simulink model "Converter_stable"  (R2021b)
settings: Solver=VariableStepAuto  StartTime=0.0  StopTime=1  FixedStep=Ts  MaxStep=Ts  RelTol=1e-3  EnableMultiTasking=on
PreLoadFcn:
  | Ts=5e-6;
  | deci=20;
InitFcn:
  | Ts=5e-6;
  | deci=20;
undefined symbols (not defined in the file): DiscIntNeverNeededParam, sps
libraries: powerlib_extras x6, spsFirstOrderFilterLib x5, spsThreePhaseSeriesRLCBranchLib x5, spsThreePhaseVIMeasurementLib x3, spsabctodq0Lib x3, spsGroundLib x3, spsSeriesRLCBranchLib x3, spsStairGeneratorLib x2, spsVoltageMeasurementLib x2, spsThreePhaseProgrammableVoltageSourceLib x2, dspsigops x1, spsdq0toabcLib x1
Description:
  | Copyright 2013-2015 Ruan Jiayang, Tsinghua Univ.
settings Model: Creator=XiaoLei  LastModifiedBy=Legend
settings DataIOCC: InitialState=xInit  LimitDataPoints=on  SaveFinalState=on  SaveFormat=StructureWithTime  SignalLoggingSaveFormat=ModelDataLogs  SaveOutput=off  SignalLogging=off  SaveTime=off  ReturnWorkspaceOutputs=off
settings OptimizationCC: ExpressionDepthLimit=2147483647  InitFltsAndDblsToZero=on  LifeSpan=inf
settings DebuggingCC: SaveWithParameterizedLinksMsg=none  UnderspecifiedInitializationDetection=Classic  MergeDetectMultiDrivingBlocksExec=none  SignalResolutionControl=TryResolveAllWithWarning  SolverPrmCheckMsg=warning  MultiTaskDSMMsg=warning  MultiTaskCondExecSysMsg=none  FcnCallInpInsideContextMsg=warning  UnconnectedInputMsg=none  UnconnectedOutputMsg=none  UnconnectedLineMsg=none  StateNameClashWarn=warning  SFUnexpectedBacktrackingDiag=warning  SFNoUnconditionalDefaultTransitionDiag=warning  SFMachineParentedDataDiag=warning  ArithmeticOperatorsInVariantConditions=warning
settings HardwareCC: ProdBitPerPointer=32  ProdBitPerSizeT=32  ProdBitPerPtrDiffT=32  ProdLargestAtomicFloat=None  ProdIntDivRoundTo=Undefined  ProdEndianess=Unspecified  ProdWordSize=32  ProdHWDeviceType=32-bit Generic
settings ModelReferenceCC: PropagateSignalLabelsOutOfModel=off
settings SFSimCC: SimUseLocalCustomCode=off  SimParseCustomCode=off  CustomCodeUndefinedFunction=UseInterfaceOnly
settings RTWCC: RTWUseLocalCustomCode=off
settings CodeAppCC: StateflowObjectComments=on
settings GRTTargetCC: TargetFcnLib=ansi_tfl_tmw.mat  TargetLangStandard=C89/C90 (ANSI)  CombineOutputUpdateFcns=off  GRTInterface=on
settings ConfigComp: CovMetricSettings=dw  CovSaveCumulativeToWorkspaceVar=on  CovSaveSingleToWorkspaceVar=on  CovExternalEMLEnable=off
settings SimscapeCC: SimscapeNormalizeSystem=off

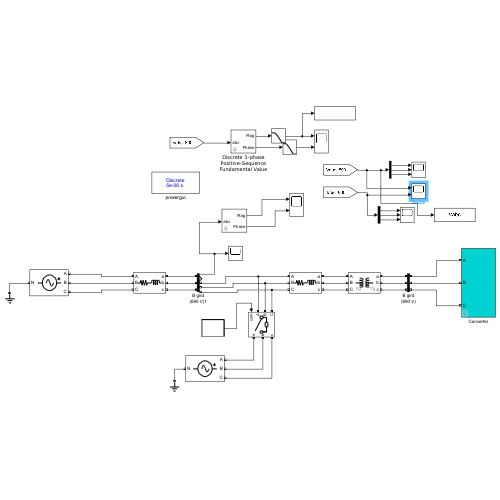
[thumbnail: Simulink's stored preview of the top-level diagram]
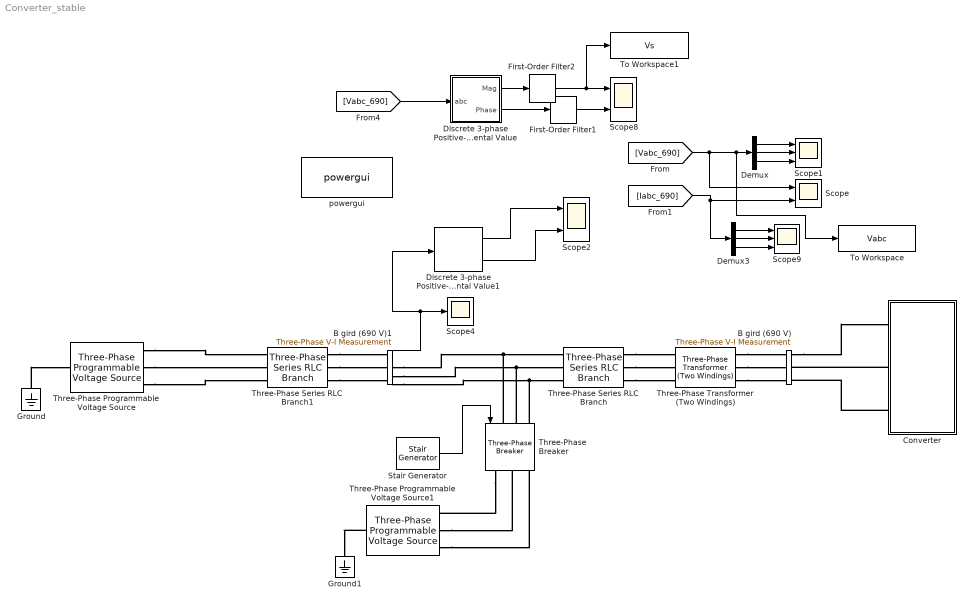
== system Converter_stable ==
  B gird (690 V) : spsThreePhaseVIMeasurementLib/Three-Phase V-I Measurement  VoltageMeasurement=phase-to-ground  SetLabelV=on  LabelV=Vabc_690  Vpu=on  VpuLL=off  CurrentMeasurement=yes  SetLabelI=on  LabelI=Iabc_690  Ipu=on  Pbase=0.5e6*0.9  Vbase=380  OutputType=Complex  PhasorSimulation=off  PSBequivalent=0
  B gird (690 V)1 : spsThreePhaseVIMeasurementLib/Three-Phase V-I Measurement  VoltageMeasurement=phase-to-ground  SetLabelV=off  LabelV=Vabc_690  Vpu=on  VpuLL=off  CurrentMeasurement=yes  SetLabelI=off  LabelI=Iabc_690  Ipu=on  Pbase=0.5e6  Vbase=10e3  OutputType=Complex  PhasorSimulation=off  PSBequivalent=0
  Converter : Subsystem  mask{Nb_wt=1, Vnom=690, Pnom1=1.5e6, Fnom=50, RL_grid=[0.01 0.25], CDC_link1=10000e-6*5, Vdc_nom=1200, Np=123, Fb_time_const=0.005, K1=[15 25 15 50/2], K2=[40 500 2 10], K3=[0.5 15], K4=0}
      mask prompts: Nb_wt "Number of wind turbines"; Vnom "Rated L-L Voltage(V)"; Pnom1 "Rated Power(VA)"; Fnom "Rated Frequency(Hz)"; RL_grid "Grid-side coupling impedance(p.u.)"; CDC_link1 "DC bus capitance (F)"; Vdc_nom "DC capacitor voltage(V)"; Np "Number of pole pairs"; Fb_time_const "Feed back time constant(s)"; K1 "rotor-side Id & Iq PID"; K2 "grid-side Vdc & Vdq PID"; K3 "rotor-side Pm PID"; K4 "gird-side Qref PID"
      mask init:
      | R_RL=RL_grid(1);
      | L_RL=RL_grid(2);
      | CDC_link=CDC_link1*Nb_wt;
      | Pnom=Pnom1*Nb_wt;
      | Inom=Pnom/sqrt(3)/Vnom;
      | Znom=Vnom/sqrt(3)/Inom;
      | Lnom=Znom/2/pi/Fnom;
      | Flux_nom=sqrt(2/3)*Vnom/2/pi/Fnom;
      | Rs_pu= 0.0034;
      | Ldq_pu= 0.352;
      | Rs=Rs_pu*Znom
      | Ldq=Ldq_pu*Lnom
      | Flux_pu=1.0017;
      | % H=0.685+4.32;
      | J_pu=0.1427/5;
      | Jnom=(2*pi*Fnom/Np)^(-2)*Pnom;
      | J=J_pu*Jnom;
      | % J=35000;%(2*pi*Fnom/Np)^(-2)*2*H*Pnom
      | Flux=Flux_pu*Flux_nom;
      | Vw_rated=11;%额定风速
      | Wr_rated=2.55;%额定转速
      | Radius=sqrt(Pnom1*2/1.225/pi/0.48/Vw_rated^3) %1.1225 is the air density, 0.44 is the maximum wind conversion rate
      | Kratio=8.119*Vw_rated/Radius/Wr_rated; %8.119 is the optimal  tip speed ratio
  Demux : Demux  Outputs=3
  Demux3 : Demux  Outputs=3
  Discrete 3-phase Positive-Sequence Fundamental Value : Subsystem  AncestorBlock=|  DialogController=POWERSYS.PowerSysDialog  mask(Discrete 3-phase Positive-sequence fundamental value){Freq=50, Par_Init=[0 0], Ts=Ts}
      | powerlib_extras/Discrete
      | Measurements/Discrete 3-phase
      | Positive-Sequence
      | Fundamental Value
      mask prompts: Freq "Fundamental frequency (Hz):"; Par_Init "Initial input (positive component): [ Mag  Phase(degrees) ]"; Ts "Sample time:"
      mask help:
      | Compute the positive-sequence component of the input signal at the given fundamental frequency. The input is set of three balanced or unbalanced signals which may contain harmonics.
      |
      | The two outputs return respectively the magnitude (same units as the input signal) and phase (in degrees) of the fundamental.
      |
      | For the first cycle of simulation, the outputs are held constant to the values specified by the Initial input parameter.
      mask init:
      | SamplesPerCycle=1/Freq/Ts;
      | RoundSamplesPerCycle=round(SamplesPerCycle);
      | Delay=RoundSamplesPerCycle*Ts - Ts/2;
      | Correction=SamplesPerCycle/RoundSamplesPerCycle - 1;
      | Real_Init=Par_Init(1)*cos(pi/180*Par_Init(2));
      | Imag_Init=Par_Init(1)*sin(pi/180*Par_Init(2));
      | power_initmask();
      mask Help: This block is part of a subset of blocks in the Extras library that does not have documentation associated with it, other than the block mask description.
      mask Display: disp('')
  Discrete 3-phase Positive-Sequence Fundamental Value1 : powerlib_extras/Discrete Measurements/Discrete 3-phase Positive-Sequence Fundamental Value  Freq=50  Par_Init=[0 0]  Ts=Ts
      settings: SourceProductBaseCode=PS
  First-Order Filter1 : spsFirstOrderFilterLib/First-Order Filter  FilterType=Lowpass  Tc=10e-3  Ts=0  Initialize=on  Vac_Init=[0, 0, 60]  Vdc_Init=0  PlotResponse=off  FreqRange="[0,  200,  1]"
  First-Order Filter2 : spsFirstOrderFilterLib/First-Order Filter  FilterType=Lowpass  Tc=5e-4  Ts=0  Initialize=on  Vac_Init=[0, 0, 60]  Vdc_Init=0  PlotResponse=off  FreqRange="[0,  200,  1]"
  Ground : spsGroundLib/Ground  LConnTagsString=a
  Ground1 : spsGroundLib/Ground  LConnTagsString=a
  Scope : Scope  NumInputPorts=2
  Scope1 : Scope  NumInputPorts=3
  Scope2 : Scope  NumInputPorts=2
  Scope4 : Scope
  Scope8 : Scope  NumInputPorts=2
  Scope9 : Scope  NumInputPorts=3
  Stair Generator : spsStairGeneratorLib/Stair Generator  t=[0, 0.6, 1.225]  e="[0, 1,  0]"  Ts=0
  Three-Phase Programmable Voltage Source : spsThreePhaseProgrammableVoltageSourceLib/Three-Phase Programmable Voltage Source  PositiveSequence=[10e3 0 50]  VariationEntity=None  VariationType=Table of time-amplitude pairs  VariationTypeAlt=Step  VariationStep=0.5  VariationRate=10  VariationMagnitude=0.3  VariationFrequency=2  VariationTiming=[1 2]  VariationPhaseA=off  Amplitudes=[1 0.15 1.0]  TimeValues=[0 0.6 2]  HarmonicGeneration=off  HarmonicA=[3 0.2 -25 0]  HarmonicB=[2 0.15 35 2]  Timing="[0.05  3]"  BusType=swing  Pref=0  Qref=0  Qmin=-inf  Qmax=inf
  Three-Phase Programmable Voltage Source1 : spsThreePhaseProgrammableVoltageSourceLib/Three-Phase Programmable Voltage Source  PositiveSequence=[0.2*10e3 -90 50]  VariationEntity=None  VariationType=Table of time-amplitude pairs  VariationTypeAlt=Step  VariationStep=0.5  VariationRate=10  VariationMagnitude=0.3  VariationFrequency=2  VariationTiming=[1 2]  VariationPhaseA=off  Amplitudes=[1 0.15 1.0]  TimeValues=[0 0.6 2]  HarmonicGeneration=off  HarmonicA=[3 0.2 -25 0]  HarmonicB=[2 0.15 35 2]  Timing="[0.05  3]"  BusType=swing  Pref=0  Qref=0  Qmin=-inf  Qmax=inf
  Three-Phase Series RLC Branch : spsThreePhaseSeriesRLCBranchLib/Three-Phase Series RLC Branch  LConnTagsString=A|B|C  RConnTagsString=A|B|C  BranchType=RL  Resistance=0.1*10*10/0.5  Inductance=0.33*10*10/0.5/314  Capacitance=1e-6  Measurements=None
  Three-Phase Series RLC Branch1 : spsThreePhaseSeriesRLCBranchLib/Three-Phase Series RLC Branch  LConnTagsString=A|B|C  RConnTagsString=A|B|C  BranchType=RL  Resistance=0.015*10*10/0.5  Inductance=0.15*10*10/0.5/314  Capacitance=1e-6  Measurements=None
  Three-Phase Transformer (Two Windings) : spsThreePhaseTransformerTwoWindingsLib/Three-Phase Transformer (Two Windings)  Winding1Connection=Yg  Winding2Connection=Yg  CoreType=Three single-phase transformers  SetSaturation=off  Hysteresis=off  DataFile='hysteresis'  SetInitialFlux=off  Measurements=None  UNITS=pu  NominalPower=[ 0.5e6 , 50 ]  Winding1=[ 10.5e3 , 0.0002 , 0.01 ]  Winding2=[ 0.38e3 , 0.0002 , 0.01 ]  Rm=500  Lm=500  L0=0.5  Saturation=[ 0,0 ; 0.0024,1.2 ; 1.0,1.52 ]  InitialFluxes=[ 0.8 , -0.8 , 0.7 ]  BreakLoop=off  DiscreteSolver=Trapezoidal iterative  DataType=off  TransfoNumber=1
  Three-Phase Breaker : spsThreePhaseBreakerLib/Three-Phase Breaker  InitialState=open  SwitchA=on  SwitchB=on  SwitchC=on  SwitchTimes="[1/60  5/60]"  External=on  BreakerResistance=0.00001  SnubberResistance=1e6  SnubberCapacitance=inf  Measurements=None
  To Workspace : ToWorkspace  VariableName=Vabc  SaveFormat=Timeseries  SampleTime=-1
  To Workspace1 : ToWorkspace  VariableName=Vs  SaveFormat=Timeseries  SampleTime=-1
  powergui : spspowerguiLib/powergui  SimulationMode=Discrete  SampleTime=Ts  frequency=50  Iterations=50  frequencyindice=0  Pbase=100e6  ErrMax=1e-4  UnitsV=kV  UnitsW=MW  buscounter=0  FunctionMessages=off  echomessages=off  EnableUseOfTLC=off  CurrentSourceSwitches=off  DisableSnubberDevices=off  DisableRonSwitches=off  DisableVfSwitches=off  DisplayEquations=off  AutomaticDiscreteSolvers=off  SolverType=Tustin/Backward Euler (TBE)  Interpol=off  ExternalGateDelay=off  methode=off  Ts=0  x0status=blocks  SPID=off  SwTol=0  HookPort=off  NonlinearTolerance=1e-4  nMaxIteration=100  ContinueOnMaxIteration=off  RestoreLinks=warning  ResistiveCurrentMeasurement=off  Frange=[0:2:500]  Ylog=off  Xlog=on  ShowGrid=off  save=off  variable=ZData  structure=Isabc  ZoomFFT=off  StartTime=1.29  cycles=2  DisplayStyle=1  fundamental=50  FreqAxis=off  MaxFrequency=1000  frequencyindicesteady=1  RmsSteady=1  display=off
  wires:
  [Vabc_690] -> Scope/1, To Workspace/1, Demux/1
  Demux/1 -> Scope1/1
  Demux/2 -> Scope1/2
  Demux/3 -> Scope1/3
  [Vabc_690] -> Discrete 3-phase Positive-Sequence Fundamental Value/1(abc)
  Discrete 3-phase Positive-Sequence Fundamental Value/2(Phase) -> First-Order Filter1/1
  Demux3/3 -> Scope9/3
  Demux3/2 -> Scope9/2
  Demux3/1 -> Scope9/1
  [Iabc_690] -> Demux3/1, Scope/2
  B gird (690 V)1/1 -> Scope4/1, Discrete 3-phase Positive-Sequence Fundamental Value1/1
  Discrete 3-phase Positive-Sequence Fundamental Value1/2 -> Scope2/2
  Discrete 3-phase Positive-Sequence Fundamental Value1/1 -> Scope2/1
  Stair Generator/1 -> Three-Phase Breaker/1
  Discrete 3-phase Positive-Sequence Fundamental Value/1(Mag) -> First-Order Filter2/1
  First-Order Filter1/1 -> Scope8/2
  First-Order Filter2/1 -> To Workspace1/1, Scope8/1
  connections:
  B gird (690 V)/RConn1 -- Converter/LConn1
  Converter/LConn2 -- B gird (690 V)/RConn2
  Converter/LConn3 -- B gird (690 V)/RConn3
  Ground/LConn1 -- Three-Phase Programmable Voltage Source/LConn1
  Three-Phase Series RLC Branch/RConn1 -- Three-Phase Transformer (Two Windings)/LConn1
  Three-Phase Series RLC Branch/RConn2 -- Three-Phase Transformer (Two Windings)/LConn2
  Three-Phase Series RLC Branch/RConn3 -- Three-Phase Transformer (Two Windings)/LConn3
  B gird (690 V)1/RConn1 -- Three-Phase Breaker/LConn1 -- Three-Phase Series RLC Branch/LConn1
  B gird (690 V)1/RConn2 -- Three-Phase Breaker/LConn2 -- Three-Phase Series RLC Branch/LConn2
  B gird (690 V)1/RConn3 -- Three-Phase Breaker/LConn3 -- Three-Phase Series RLC Branch/LConn3
  Three-Phase Programmable Voltage Source/RConn1 -- Three-Phase Series RLC Branch1/LConn1
  Three-Phase Programmable Voltage Source/RConn2 -- Three-Phase Series RLC Branch1/LConn2
  Three-Phase Programmable Voltage Source/RConn3 -- Three-Phase Series RLC Branch1/LConn3
  Three-Phase Transformer (Two Windings)/RConn1 -- B gird (690 V)/LConn1
  Three-Phase Transformer (Two Windings)/RConn2 -- B gird (690 V)/LConn2
  Three-Phase Transformer (Two Windings)/RConn3 -- B gird (690 V)/LConn3
  Three-Phase Series RLC Branch1/RConn1 -- B gird (690 V)1/LConn1
  Three-Phase Series RLC Branch1/RConn2 -- B gird (690 V)1/LConn2
  Three-Phase Series RLC Branch1/RConn3 -- B gird (690 V)1/LConn3
  Three-Phase Programmable Voltage Source1/RConn2 -- Three-Phase Breaker/RConn2
  Three-Phase Breaker/RConn1 -- Three-Phase Programmable Voltage Source1/RConn1
  Three-Phase Programmable Voltage Source1/RConn3 -- Three-Phase Breaker/RConn3
  Three-Phase Programmable Voltage Source1/LConn1 -- Ground1/LConn1

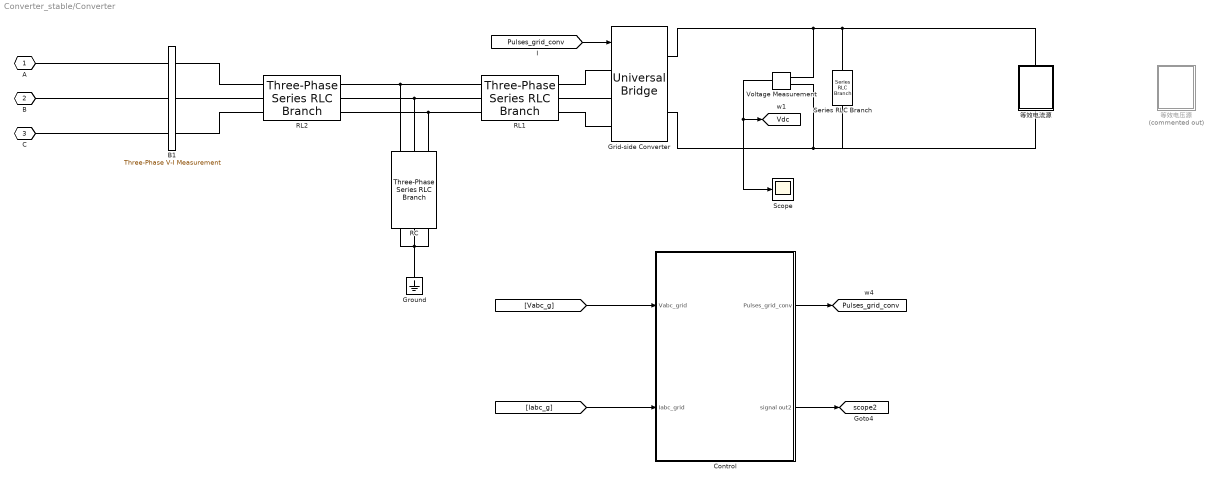
== system Converter_stable/Converter ==
  B1 : spsThreePhaseVIMeasurementLib/Three-Phase V-I Measurement  VoltageMeasurement=phase-to-ground  SetLabelV=on  LabelV=Vabc_g  Vpu=on  VpuLL=off  CurrentMeasurement=yes  SetLabelI=on  LabelI=Iabc_g  Ipu=on  Pbase=0.5e6  Vbase=380  OutputType=Complex  PhasorSimulation=off  PSBequivalent=0
  Control : Subsystem
  Grid-side Converter : spsUniversalBridgeLib/Universal Bridge  Arms=3  SnubberResistance=1e6  SnubberCapacitance=inf  Device=IGBT / Diodes  Ron=1e-7  Lon=0  ForwardVoltages="[  0  0  ]"  ForwardVoltage=0  GTOparameters=[ 10e-6 , 20e-6 ]  IGBTparameters=[0 , 0]  Measurements=None  Measurements_2=None  converterType=Rectifier
  Ground : spsGroundLib/Ground  LConnTagsString=a
  RC : spsThreePhaseSeriesRLCBranchLib/Three-Phase Series RLC Branch  LConnTagsString=A|B|C  RConnTagsString=A|B|C  BranchType=RC  Resistance=1.5  Inductance=L_RL*Vnom^2/Pnom/(2*pi*Fnom)  Capacitance=1000e-6  Measurements=None
  RL1 : spsThreePhaseSeriesRLCBranchLib/Three-Phase Series RLC Branch  LConnTagsString=A|B|C  RConnTagsString=A|B|C  BranchType=RL  Resistance=0.0002  Inductance=0.7/1000  Capacitance=1.0  Measurements=None
  RL2 : spsThreePhaseSeriesRLCBranchLib/Three-Phase Series RLC Branch  LConnTagsString=A|B|C  RConnTagsString=A|B|C  BranchType=RL  Resistance=0.0001  Inductance=0.3/1000  Capacitance=1.0  Measurements=None
  Scope : Scope
  Series RLC Branch : spsSeriesRLCBranchLib/Series RLC Branch  LConnTagsString=__new0  RConnTagsString=__new0  BranchType=C  Resistance=1  Inductance=1e-3  SetiL0=off  InitialCurrent=0  Capacitance=10000e-6  Setx0=on  InitialVoltage=790  Measurements=None
  Voltage Measurement : spsVoltageMeasurementLib/Voltage Measurement  PhasorSimulation=off  OutputType=Complex  PSBequivalent=0
  等效电压源 : Subsystem  Commented=on
  等效电流源 : Subsystem
  A : PMIOPort  Tag=PMCPort  Side=Left
  B : PMIOPort  Tag=PMCPort  Port=2  Side=Left
  C : PMIOPort  Tag=PMCPort  Port=3  Side=Left
  tag scope: Pulses_grid_conv=global, Vdc=global, scope2=global
  wires:
  [Pulses_grid_conv] -> Grid-side Converter/1
  Control/1(Pulses_grid_conv) -> [Pulses_grid_conv]
  Control/2(signal out2) -> [scope2]
  [Vabc_g] -> Control/1(Vabc_grid)
  [Iabc_g] -> Control/2(Iabc_grid)
  Voltage Measurement/1 -> Scope/1, [Vdc]
  connections:
  RL1/RConn1 -- Grid-side Converter/LConn1
  RL1/RConn2 -- Grid-side Converter/LConn2
  RL1/RConn3 -- Grid-side Converter/LConn3
  C/RConn1 -- B1/LConn3
  B1/LConn1 -- A/RConn1
  B1/LConn2 -- B/RConn1
  Ground/LConn1 -- RC/RConn2 -- RC/RConn3 -- RC/RConn1
  B1/RConn1 -- RL2/LConn1
  B1/RConn2 -- RL2/LConn2
  B1/RConn3 -- RL2/LConn3
  RL2/RConn1 -- RL1/LConn1 -- RC/LConn1
  RL2/RConn2 -- RL1/LConn2 -- RC/LConn2
  RL2/RConn3 -- RC/LConn3 -- RL1/LConn3
  Series RLC Branch/LConn1 -- 等效电流源/RConn1 -- Voltage Measurement/LConn1 -- Grid-side Converter/RConn1
  Grid-side Converter/RConn2 -- 等效电流源/LConn1 -- Series RLC Branch/RConn1 -- Voltage Measurement/LConn2

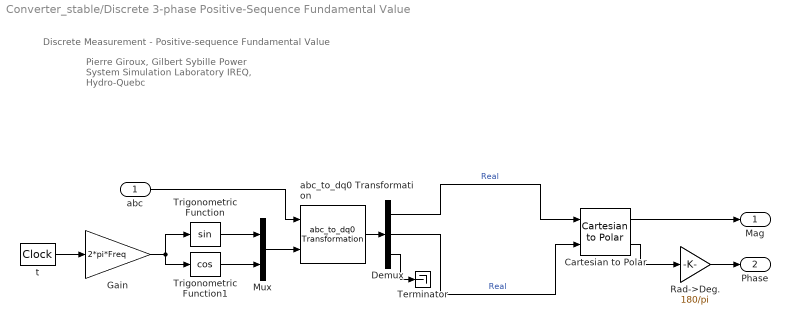
== system Converter_stable/Discrete 3-phase Positive-Sequence Fundamental Value ==
  note: Pierre Giroux, Gilbert Sybille
      | Power System Simulation Laboratory
      | IREQ, Hydro-Quebc
  note: Discrete Measurement - Positive-sequence Fundamental Value
  abc : Inport  PortDimensions=3
  Cartesian to Polar : simulink_extras/Transformations/Cartesian to Polar
  Demux : Demux  Outputs=3
      settings: DisplayOption=none
  Gain : Gain  Gain=2*pi*Freq  SaturateOnIntegerOverflow=on  OutDataTypeStr=Inherit: Same as input  ParamDataTypeStr=Inherit: Same as input
  Mux : Mux  Inputs=2
  Rad->Deg. : Gain  Gain=180/pi  SaturateOnIntegerOverflow=on  OutDataTypeStr=Inherit: Same as input  ParamDataTypeStr=Inherit: Same as input
  Terminator : Terminator
  Trigonometric Function : Trigonometry
  Trigonometric Function1 : Trigonometry  Operator=cos
  abc_to_dq0 Transformation : powerlib_extras/Measurements/abc_to_dq0 Transformation
      settings: SourceProductBaseCode=PS
  t : DigitalClock  SampleTime=Ts
  Mag : Outport  VectorParamsAs1DForOutWhenUnconnected=off
  Phase : Outport  Port=2  VectorParamsAs1DForOutWhenUnconnected=off
  wires:
  Cartesian to Polar/2 -> Rad->Deg./1
  Cartesian to Polar/1 -> Mag/1
  Gain/1 -> Trigonometric Function1/1, Trigonometric Function/1
  t/1 -> Gain/1
  abc/1 -> abc_to_dq0 Transformation/1
  Mux/1 -> abc_to_dq0 Transformation/2
  Demux/1 -> Cartesian to Polar/1  "Real"
  Rad->Deg./1 -> Phase/1
  Demux/2 -> Cartesian to Polar/2  "Real"
  abc_to_dq0 Transformation/1 -> Demux/1
  Demux/3 -> Terminator/1
  Trigonometric Function/1 -> Mux/1
  Trigonometric Function1/1 -> Mux/2

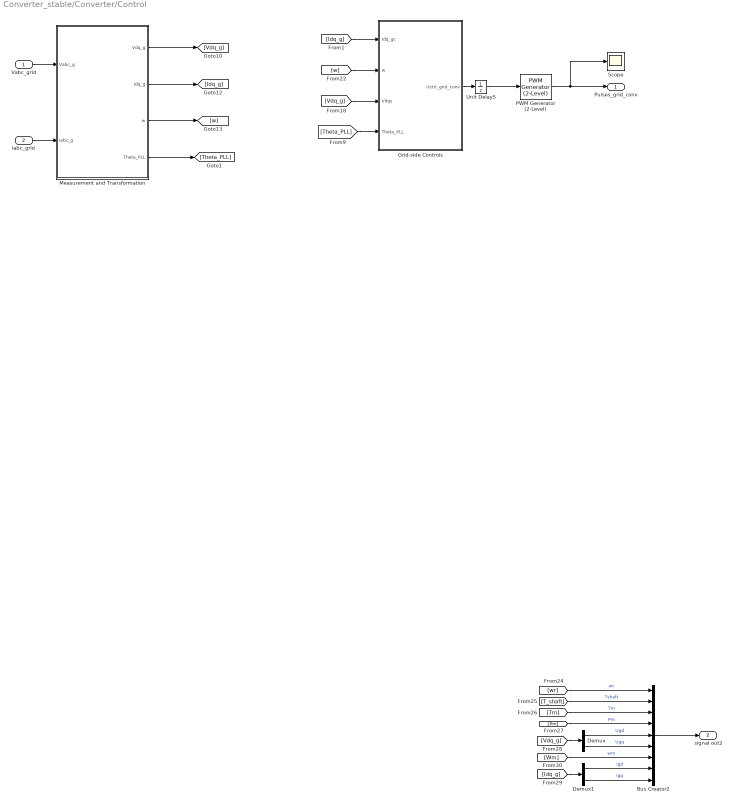
== system Converter_stable/Converter/Control ==
  Vabc_grid : Inport
  Iabc_grid : Inport  Port=2
  Bus Creator2 : BusCreator  Inputs=9
  Demux : Demux  Outputs=2
  Demux1 : Demux  Outputs=2
  Grid-side Controls : Subsystem
  Measurement and Transformation : Subsystem
  PWM Generator (2-Level) : spsPWMGenerator2LevelLib/PWM Generator (2-Level)  ModulatorType=Three-phase bridge (6 pulses)  ModulatorMode=Unsynchronized  Fc=3000  Pc=90  nF=27  MinMax="[ -1  1 ]"  SamplingTechnique=Natural  ModulatingSignals=off  m=0.8  Freq=60  Phase=0  Ts=Ts  ShowCarrierOutport=off
  Scope : Scope
  Unit Delay5 : UnitDelay  SampleTime=Ts  HasFrameUpgradeWarning=on
  Pulses_grid_conv : Outport
  signal out2 : Outport  Port=2
  wires:
  Measurement and Transformation/3(w) -> [w]
  Measurement and Transformation/2(Idq_g) -> [Idq_g]
  Measurement and Transformation/1(Vdq_g) -> [Vdq_g]
  Iabc_grid/1 -> Measurement and Transformation/2(Iabc_g)
  Vabc_grid/1 -> Measurement and Transformation/1(Vabc_g)
  Measurement and Transformation/4(Theta_PLL) -> [Theta_PLL]
  [Vdq_g] -> Grid-side Controls/3(Vdqs)
  [w] -> Grid-side Controls/2(w)
  [Idq_g] -> Grid-side Controls/1(Idq_gc)
  [Theta_PLL] -> Grid-side Controls/4(Theta_PLL)
  [wr] -> Bus Creator2/1  "wr"
  [T_shaft] -> Bus Creator2/2  "Tshaft"
  [Tm] -> Bus Creator2/3  "Tm"
  [Pm] -> Bus Creator2/4  "Pm"
  Bus Creator2/1 -> signal out2/1
  [Wm] -> Bus Creator2/7  "wm"
  [Vdq_g] -> Demux/1
  [Idq_g] -> Demux1/1
  Demux/1 -> Bus Creator2/5  "Ugd"
  Demux/2 -> Bus Creator2/6  "Ugq"
  Demux1/1 -> Bus Creator2/8  "Igd"
  Demux1/2 -> Bus Creator2/9  "Igq"
  Grid-side Controls/1(Uctrl_grid_conv) -> Unit Delay5/1
  Unit Delay5/1 -> PWM Generator (2-Level)/1
  PWM Generator (2-Level)/1 -> Pulses_grid_conv/1, Scope/1

== system Converter_stable/Converter/等效电压源 ==
  DC Voltage Source : spsDCVoltageSourceLib/DC Voltage Source  Amplitude=790  Measurements=None
  Series RLC Branch1 : spsSeriesRLCBranchLib/Series RLC Branch  LConnTagsString=__new0  RConnTagsString=__new0  BranchType=R  Resistance=0.01  Inductance=1e-3  SetiL0=off  InitialCurrent=0  Capacitance=5000e-6  Setx0=on  InitialVoltage=790  Measurements=None
  Conn1 : PMIOPort  Side=Right
  - : PMIOPort  Port=2  Side=Left
  connections:
  Series RLC Branch1/LConn1 -- DC Voltage Source/RConn1
  DC Voltage Source/LConn1 -- -/RConn1
  Series RLC Branch1/RConn1 -- Conn1/RConn1

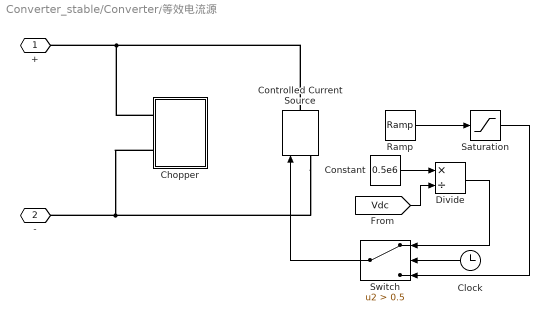
== system Converter_stable/Converter/等效电流源 ==
  Chopper : Subsystem
  Clock : Clock
  Constant : Constant  Value=0.5e6
  Controlled Current Source : spsControlledCurrentSourceLib/Controlled Current Source  Initialize=on  Source_Type=AC  Amplitude=0  Phase=0  Frequency=0  Measurements=None
  Divide : Product  Inputs=*/
  Ramp : simulink/Sources/Ramp  slope=0.5e6/790*4  start=0  InitialOutput=0
  Saturation : Saturate  UpperLimit=0.5e6/790  LowerLimit=0
  Switch : Switch  Criteria=u2 > Threshold  Threshold=0.5
  + : PMIOPort  Side=Right
  - : PMIOPort  Port=2  Side=Left
  wires:
  Divide/1 -> Switch/1
  Switch/1 -> Controlled Current Source/1
  Saturation/1 -> Switch/3
  Ramp/1 -> Saturation/1
  [Vdc] -> Divide/2
  Clock/1 -> Switch/2
  Constant/1 -> Divide/1
  connections:
  Controlled Current Source/LConn1 -- Chopper/LConn2 -- -/RConn1
  Controlled Current Source/RConn1 -- Chopper/LConn1 -- +/RConn1

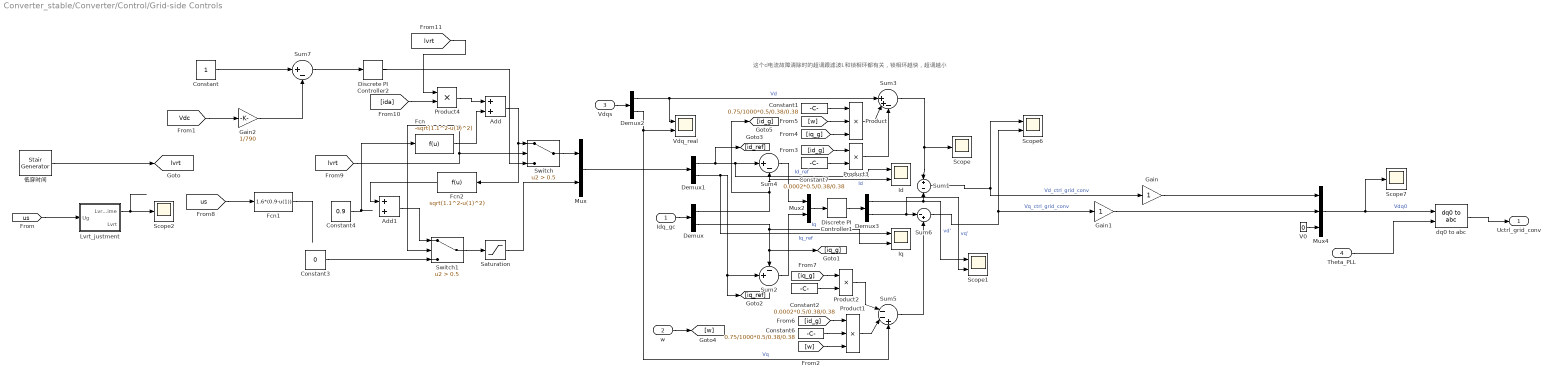
== system Converter_stable/Converter/Control/Grid-side Controls ==
  note: 这个d电流故障清除时的超调跟滤波L和锁相环都有关，锁相环越快，超调越小
  Idq_gc : Inport
  w : Inport  Port=2
  Vdqs : Inport  Port=3
  Theta_PLL : Inport  Port=4
  Add : Sum
  Add1 : Sum
  Constant : Constant
  Constant1 : Constant  Value=0.75/1000*0.5/0.38/0.38
  Constant2 : Constant  Value=0.0002*0.5/0.38/0.38
  Constant3 : Constant  Value=0
  Constant4 : Constant  Value=0.9
  Constant6 : Constant  Value=0.75/1000*0.5/0.38/0.38
  Constant7 : Constant  Value=0.0002*0.5/0.38/0.38
  Demux{,1..3} (4 alike) : Demux  Outputs=2
      settings: DisplayOption=none
  Discrete PI Controller1 : powerlib_extras/Discrete  Control Blocks/Discrete PI Controller  Kp=0.5*50  Ki=0.3*50  Par_Limits=[0.5 -0.5]*4  Init=0  Ts=Ts
  Discrete PI Controller2 : powerlib_extras/Discrete  Control Blocks/Discrete PI Controller  Kp=5  Ki=20  Par_Limits=[1.1 -1.1]  Init=0  Ts=Ts
  Fcn : Fcn  Expr=-sqrt(1.1^2-u(1)^2)
  Fcn1 : Fcn  Expr=1.6*(0.9-u(1))
  Fcn2 : Fcn  Expr=sqrt(1.1^2-u(1)^2)
  Gain : Gain
  Gain1 : Gain
  Gain2 : Gain  Gain=1/790
  Id : Scope  NumInputPorts=2
  Iq : Scope  NumInputPorts=2
  Lvrt_justment : Subsystem  mask{Th=0}
      mask prompts: Th "Hold Time"
  Mux : Mux  Inputs=2
  Mux2 : Mux  Inputs=2
  Mux4 : Mux  Inputs=3
  Product : Product  Inputs=3  InputSameDT=on  SaturateOnIntegerOverflow=on  OutDataTypeStr=Inherit: Same as first input
  Product1 : Product  Inputs=3  InputSameDT=on  SaturateOnIntegerOverflow=on  OutDataTypeStr=Inherit: Same as first input
  Product2 : Product  InputSameDT=on  SaturateOnIntegerOverflow=on  OutDataTypeStr=Inherit: Same as first input
  Product3 : Product  InputSameDT=on  SaturateOnIntegerOverflow=on  OutDataTypeStr=Inherit: Same as first input
  Product4 : Product
  Saturation : Saturate  UpperLimit=1.2
  Scope : Scope
  Scope1 : Scope  NumInputPorts=2
  Scope2 : Scope
  Scope6 : Scope  NumInputPorts=2
  Scope7 : Scope
  Sum1 : Sum  Inputs=+-  InputSameDT=on  SaturateOnIntegerOverflow=on  OutDataTypeStr=Inherit: Same as first input
  Sum2 : Sum  Inputs=-+|  InputSameDT=on  SaturateOnIntegerOverflow=on  OutDataTypeStr=Inherit: Same as first input
  Sum3 : Sum  Inputs=||++-  InputSameDT=on  SaturateOnIntegerOverflow=on  OutDataTypeStr=Inherit: Same as first input
  Sum4 : Sum  Inputs=|+-  InputSameDT=on  SaturateOnIntegerOverflow=on  OutDataTypeStr=Inherit: Same as first input
  Sum5 : Sum  Inputs=|--+  InputSameDT=on  SaturateOnIntegerOverflow=on  OutDataTypeStr=Inherit: Same as first input
  Sum6 : Sum  Inputs=|-+  InputSameDT=on  SaturateOnIntegerOverflow=on  OutDataTypeStr=Inherit: Same as first input
  Sum7 : Sum  Inputs=|+-  InputSameDT=on  SaturateOnIntegerOverflow=on  OutDataTypeStr=Inherit: Same as first input
  Switch : Switch  Criteria=u2 > Threshold  Threshold=0.5
  Switch1 : Switch  Criteria=u2 > Threshold  Threshold=0.5
  V0 : Constant  Value=0
  Vdq_real : Scope  NumInputPorts=2
  dq0 to abc : spsdq0toabcLib/dq0 to abc  Alignment=90 degrees behind phase A axis
  低穿时间 : spsStairGeneratorLib/Stair Generator  t=[0, 0.6, 1.225]  e=[0, 1, 0]  Ts=0
  Uctrl_grid_conv : Outport
  tag scope: lvrt=global
  wires:
  Sum5/1 -> Sum6/2
  Sum3/1 -> Sum1/1, Scope/1
  Demux1/1 -> [id_ref], Id/1, Sum4/1  "Id_ref"
  Demux1/2 -> Iq/1, [iq_ref], Sum2/2  "Iq_ref"
  Demux3/2 -> Scope1/2, Sum6/1  "vq'"
  Demux3/1 -> Scope1/1, Sum1/2  "vd'"
  [id_g] -> Product1/1
  [iq_g] -> Product/3
  [w] -> Product/2
  [w] -> Product1/3
  Sum2/1 -> Mux2/2
  Sum4/1 -> Mux2/1
  Demux2/2 -> Sum5/3, Vdq_real/2  "Vq"
  Product1/1 -> Sum5/2
  Product/1 -> Sum3/2
  Vdqs/1 -> Demux2/1
  Constant1/1 -> Product/1
  Demux2/1 -> Sum3/1, Vdq_real/1  "Vd"
  Mux2/1 -> Discrete PI Controller1/1
  Discrete PI Controller1/1 -> Demux3/1
  Constant6/1 -> Product1/2
  w/1 -> [w]
  V0/1 -> Mux4/3
  Mux4/1 -> dq0 to abc/1, Scope7/1  "Vdq0"
  Theta_PLL/1 -> dq0 to abc/2
  dq0 to abc/1 -> Uctrl_grid_conv/1
  Sum1/1 -> Gain/1, Scope6/1  "Vd_ctrl_grid_conv"
  Sum6/1 -> Gain1/1, Scope6/2  "Vq_ctrl_grid_conv"
  Idq_gc/1 -> Demux/1
  Demux/1 -> [id_g], Id/2, Sum4/2  "Id"
  Demux/2 -> Iq/2, [iq_g], Sum2/1  "Iq"
  Mux/1 -> Demux1/1
  Discrete PI Controller2/1 -> Switch/3
  Switch1/1 -> Saturation/1
  Fcn/1 -> Add/2
  Switch/1 -> Mux/1
  Gain/1 -> Mux4/1
  Gain1/1 -> Mux4/2
  Constant/1 -> Sum7/1
  [Vdc] -> Gain2/1
  Gain2/1 -> Sum7/2
  Constant3/1 -> Switch1/3
  [us] -> Fcn1/1
  Sum7/1 -> Discrete PI Controller2/1
  Constant2/1 -> Product2/2
  [iq_g] -> Product2/1
  Product2/1 -> Sum5/1
  [id_g] -> Product3/1
  Constant7/1 -> Product3/2
  Product3/1 -> Sum3/3
  [lvrt] -> Switch1/2, Switch/2
  Saturation/1 -> Mux/2
  低穿时间/1 -> [lvrt]
  [us] -> Lvrt_justment/1(Ug)
  Lvrt_justment/1(Lvrt_time) -> Scope2/1
  Fcn1/1 -> ?
  Add1/1 -> Switch1/1
  [ida] -> Product4/2
  Add/1 -> Fcn2/1, Switch/1
  Product4/1 -> Add/1
  [lvrt] -> Product4/1
  Constant4/1 -> Fcn/1
  Fcn2/1 -> Add1/1

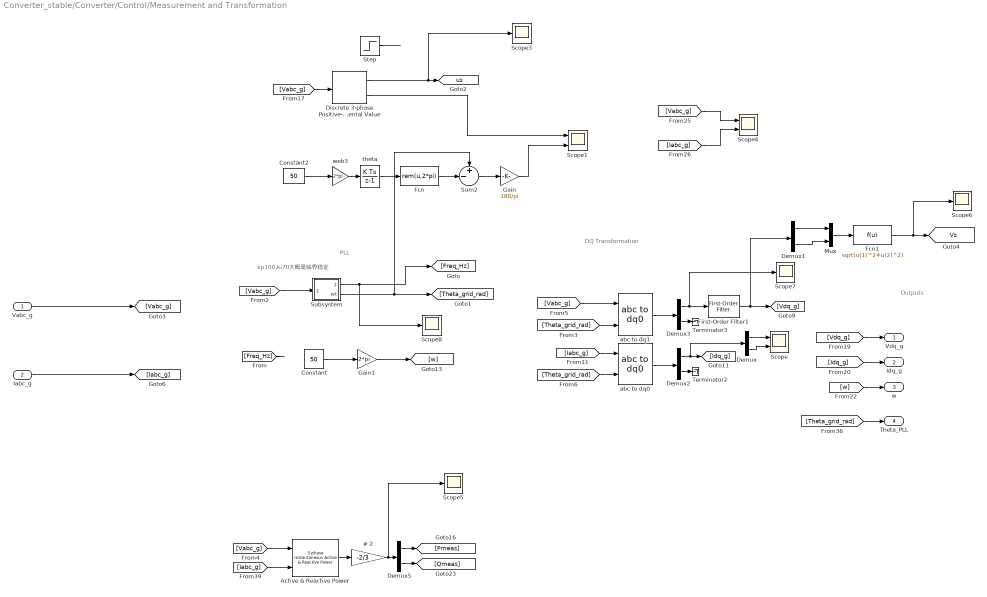
== system Converter_stable/Converter/Control/Measurement and Transformation ==
  note: kp100,ki70大概是临界稳定
  note: Outputs
  note: PLL
  note: DQ Transformation
  Vabc_g : Inport
  Iabc_g : Inport  Port=2
  # 2 : Gain  Gain=-2/3  SaturateOnIntegerOverflow=on  OutDataTypeStr=Inherit: Same as input  ParamDataTypeStr=Inherit: Same as input
  Active & Reactive Power : powerlib_extras/Measurements/3-phase  Instantaneous  Active & Reactive Power
      settings: SourceProductBaseCode=PS
  Constant : Constant  Value=50
  Constant2 : Constant  Value=50  SampleTime=Ts
  Demux : Demux  Outputs=2
  Demux1 : Demux  Outputs=2
      settings: DisplayOption=none
  Demux2 : Demux  Outputs=[2 1]
      settings: DisplayOption=none
  Demux3 : Demux  Outputs=[2 1]
      settings: DisplayOption=none
  Demux5 : Demux  Outputs=2
      settings: DisplayOption=none
  Discrete 3-phase Positive-Sequence Fundamental Value : powerlib_extras/Discrete Measurements/Discrete 3-phase Positive-Sequence Fundamental Value  Freq=50  Par_Init=[0 0]  Ts=Ts
      settings: SourceProductBaseCode=PS
  Fcn : Fcn  Expr=rem(u,2*pi)
  Fcn1 : Fcn  Expr=sqrt(u(1)^2+u(2)^2)
  First-Order Filter1 : spsFirstOrderFilterLib/First-Order Filter  FilterType=Lowpass  Tc=10e-4  Ts=0  Initialize=on  Vac_Init=[0, 0, 50]  Vdc_Init=0  PlotResponse=off  FreqRange="[0,  200,  1]"
  Gain : Gain  Gain=180/pi
  Gain1 : Gain  Gain=2*pi
  Mux : Mux  Inputs=2
  Scope : Scope  NumInputPorts=2
  Scope1 : Scope  NumInputPorts=2
  Scope{3,5..8} (5 alike) : Scope
  Scope4 : Scope  NumInputPorts=2
  Step : Step  Time=0.4  Before=0.9  After=0.32  SampleTime=0
  Subsystem : Subsystem  mask{kp=0.7, ki=60, wb=100*pi, wg=1}
  Sum2 : Sum  Inputs=+-|  InputSameDT=on  SaturateOnIntegerOverflow=on  OutDataTypeStr=Inherit: Same as first input
  Terminator2 : Terminator
  Terminator3 : Terminator
  abc to dq0 : spsabctodq0Lib/abc to dq0  Alignment=90 degrees behind phase A axis
  abc to dq1 : spsabctodq0Lib/abc to dq0  Alignment=90 degrees behind phase A axis
  theta : DiscreteIntegrator  SampleTime=Ts  ICPrevOutput=DiscIntNeverNeededParam  ICPrevScaledInput=DiscIntNeverNeededParam
  web3 : Gain  Gain=2*pi  SaturateOnIntegerOverflow=on  OutDataTypeStr=Inherit: Same as input  ParamDataTypeStr=Inherit: Same as input
  Vdq_g : Outport
  Idq_g : Outport  Port=2
  w : Outport  Port=3
  Theta_PLL : Outport  Port=4
  tag scope: Vs=global, us=global
  wires:
  Iabc_g/1 -> [Iabc_g]
  Vabc_g/1 -> [Vabc_g]
  [w] -> w/1
  [Idq_g] -> Idq_g/1
  [Vdq_g] -> Vdq_g/1
  Demux2/1 -> Demux/1, [Idq_g]
  [Iabc_g] -> abc to dq0/1
  [Theta_grid_rad] -> abc to dq0/2
  [Theta_grid_rad] -> abc to dq1/2
  [Vabc_g] -> abc to dq1/1
  [Freq_Hz] -> ?
  abc to dq0/1 -> Demux2/1
  Demux2/2 -> Terminator2/1
  abc to dq1/1 -> Demux3/1
  Demux3/2 -> Terminator3/1
  [Theta_grid_rad] -> Theta_PLL/1
  [Vabc_g] -> Active & Reactive Power/1
  [Iabc_g] -> Active & Reactive Power/2
  Demux5/1 -> [Pmeas]
  Demux5/2 -> [Qmeas]
  Active & Reactive Power/1 -> # 2/1
  # 2/1 -> Scope5/1, Demux5/1
  Demux/1 -> Scope/1
  Demux/2 -> Scope/2
  Subsystem/1(Freq) -> Scope8/1, [Freq_Hz]
  web3/1 -> theta/1
  theta/1 -> Fcn/1
  Constant2/1 -> web3/1
  Fcn/1 -> Sum2/2
  Subsystem/2(wt) -> Sum2/1, [Theta_grid_rad]
  Sum2/1 -> Gain/1
  Gain/1 -> Scope1/2
  [Vabc_g] -> Discrete 3-phase Positive-Sequence Fundamental Value/1
  [Vabc_g] -> Scope4/1
  [Iabc_g] -> Scope4/2
  [Vabc_g] -> Subsystem/1(Vabc)
  Discrete 3-phase Positive-Sequence Fundamental Value/1 -> Scope3/1, [us]
  Discrete 3-phase Positive-Sequence Fundamental Value/2 -> Scope1/1
  Step/1 -> ?
  Gain1/1 -> [w]
  Constant/1 -> Gain1/1
  Demux3/1 -> Scope7/1, First-Order Filter1/1
  First-Order Filter1/1 -> Demux1/1, [Vdq_g]
  Demux1/1 -> Mux/1
  Demux1/2 -> Mux/2
  Mux/1 -> Fcn1/1
  Fcn1/1 -> Scope6/1, [Vs]

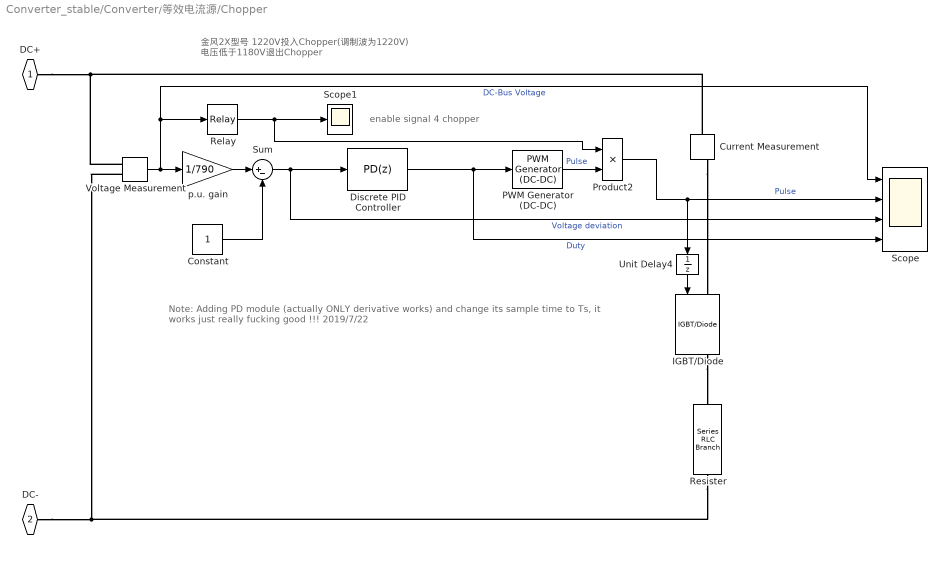
== system Converter_stable/Converter/等效电流源/Chopper ==
  note: enable signal 4 chopper
  note: 金风2X型号 1220V投入Chopper(调制波为1220V)
      | 电压低于1180V退出Chopper
  note: Note: Adding PD module (actually ONLY derivative works) and change its sample time to Ts,
      |  it works just really fucking good !!!
      | 2019/7/22
  Constant : Constant
  Current Measurement : spsCurrentMeasurementLib/Current Measurement  PhasorSimulation=off  OutputType=Complex  PSBequivalent=0
  Discrete PID Controller : slpidlib/PID Controller  Controller=PD  Form=Ideal  TimeDomain=Discrete-time  UseExternalTs=off  SampleTime=Ts  IntegratorMethod=Forward Euler  FilterMethod=Forward Euler  ControllerParametersSource=internal  P=1  I=1  D=100  UseFilter=on  N=1  TunerSelectOption=Transfer Function Based (PID Tuner App)  InitialConditionSource=internal  InitialConditionForIntegrator=0  InitialConditionForFilter=0  DifferentiatorICPrevScaledInput=0  ExternalReset=none  TrackingMode=off  Kt=1  LimitOutput=on  SatLimitsSource=internal  UpperSaturationLimit=1  LowerSaturationLimit=0  LinearizeAsGain=off  AntiWindupMode=none  Kb=1  POutMin=[]  POutMax=[]  IOutMin=[]  IOutMax=[]  DOutMin=[]  DOutMax=[]  NOutMin=[]  NOutMax=[]  SumOutMin=[]  SumOutMax=[]  SaturationOutMin=[]  SaturationOutMax=[]  PParamMin=[]  PParamMax=[]  IParamMin=[]  IParamMax=[]  DParamMin=[]  DParamMax=[]  NParamMin=[]  NParamMax=[]  KbParamMin=[]  KbParamMax=[]  KtParamMin=[]  KtParamMax=[]  KbOutMin=[]  KbOutMax=[]  KtOutMin=[]  KtOutMax=[]  IntegratorOutMin=[]  IntegratorOutMax=[]  FilterOutMin=[]  FilterOutMax=[]  SumI1OutMin=[]  SumI1OutMax=[]  SumI2OutMin=[]  SumI2OutMax=[]  SumI3OutMin=[]  SumI3OutMax=[]  SumI4OutMin=[]  SumI4OutMax=[]  SumDOutMin=[]  SumDOutMax=[]  DifferentiatorOutMin=[]  DifferentiatorOutMax=[]  FilterDiffOutCoefMin=[]  FilterDiffOutCoefMax=[]  ReciprocalOutMin=[]  ReciprocalOutMax=[]  SumDenOutMin=[]  SumDenOutMax=[]  SumNumOutMin=[]  SumNumOutMax=[]  DivideOutMin=[]  DivideOutMax=[]  UdiffTsProdOutMin=[]  UdiffTsProdOutMax=[]  NTsProdOutMin=[]  NTsProdOutMax=[]  UintegralTsProdOutMin=[]  UintegralTsProdOutMax=[]  UngainTsProdOutMin=[]  UngainTsProdOutMax=[]  IntegratorContinuousStateAttributes=''  IntegratorStateMustResolveToSignalObject=off  IntegratorRTWStateStorageClass=Auto  FilterContinuousStateAttributes=''  FilterStateMustResolveToSignalObject=off  FilterRTWStateStorageClass=Auto  ParallelPVariant=Passthrough  IdealPVariant=InternalParameters  IVariant=Disabled  DVariant=InternalParameters  IntegratorVariant=Disabled  SatVariant=Enabled  AWVariant=Disabled  PCopyVariant=Disabled  TRVariant=Disabled  FdbkBlocksVariant=Forward  IdealPFdbkVariant=Disabled  SatFdbkVariant=Disabled  DerivativeFilterVariant=ForwardEulerFilter  NVariant=InternalParameters  NCopyVariant=Disabled  FilterICVariant=InternalICsFilter  IntegratorICVariant=Disabled  ExternalResetVariant=Disabled  TRSumVariant=Passthrough  SumFdbkVariant=Disabled  SumVariant=Sum_PD  TsampFilterVariant=InternalTs  TsampNgainVariant=Passthrough  TsampIntegralVariant=Disabled_SignalSpec  ExternalSaturationOutDataTypeStr=Inherit: Same as second input
  IGBT/Diode : spsIGBTDiodeLib/IGBT//Diode  Ron=1e-3  Rs=1e5  Cs=inf  Measurements=on
  PWM Generator (DC-DC) : spsPWMGeneratorDCDCLib/PWM Generator (DC-DC)  Fsw=1e3  Ts=0
  Product2 : Product  InputSameDT=on  SaturateOnIntegerOverflow=on  OutDataTypeStr=Inherit: Same as first input
  Relay : Relay  OnSwitchValue=900  OffSwitchValue=880
  Resister : spsSeriesRLCBranchLib/Series RLC Branch  LConnTagsString=__new0  RConnTagsString=__new0  BranchType=R  Resistance=0.1  Inductance=1e-3  SetiL0=off  InitialCurrent=0  Capacitance=1e-6  Setx0=off  InitialVoltage=0  Measurements=None
  Scope : Scope  NumInputPorts=4
  Scope1 : Scope
  Sum : Sum  Inputs=|+-
  Unit Delay4 : UnitDelay  SampleTime=Ts  HasFrameUpgradeWarning=on
  Voltage Measurement : spsVoltageMeasurementLib/Voltage Measurement  PhasorSimulation=off  OutputType=Complex  PSBequivalent=0
  p.u. gain : Gain  Gain=1/790
  DC+ : PMIOPort  Side=Left
  DC- : PMIOPort  Port=2  Side=Left
  wires:
  Unit Delay4/1 -> IGBT/Diode/1
  Product2/1 -> Unit Delay4/1, Scope/2  "Pulse"
  Voltage Measurement/1 -> Scope/1, Relay/1, p.u. gain/1  "DC-Bus Voltage"
  Sum/1 -> Discrete PID Controller/1, Scope/3  "Voltage deviation"
  Discrete PID Controller/1 -> Scope/4, PWM Generator (DC-DC)/1  "Duty"
  Relay/1 -> Product2/1, Scope1/1
  p.u. gain/1 -> Sum/1
  Constant/1 -> Sum/2
  PWM Generator (DC-DC)/1 -> Product2/2  "Pulse"
  connections:
  Voltage Measurement/LConn1 -- DC+/RConn1 -- Current Measurement/LConn1
  Resister/RConn1 -- Voltage Measurement/LConn2 -- DC-/RConn1
  Current Measurement/RConn1 -- IGBT/Diode/LConn1
  IGBT/Diode/RConn1 -- Resister/LConn1

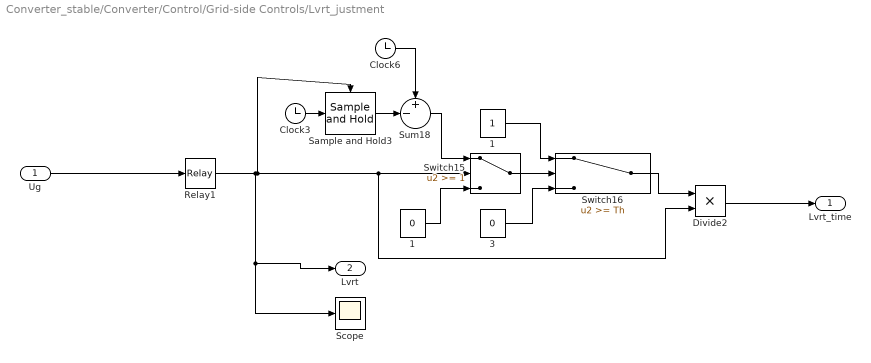
== system Converter_stable/Converter/Control/Grid-side Controls/Lvrt_justment ==
  Ug : Inport
  " 1" : Constant  Value=0
  " 3" : Constant  Value=0
  " 1" : Constant
  Clock3 : Clock
  Clock6 : Clock
  Divide2 : Product  Inputs=**
  Relay1 : Relay  OnSwitchValue=0.89  OffSwitchValue=0.87  OnOutputValue=0  OffOutputValue=1
  Sample and Hold3 : dspsigops/Sample and Hold  trig=Rising edge  initCond=0  latchinput=off
  Scope : Scope
  Sum18 : Sum  Inputs=+-|  InputSameDT=on  SaturateOnIntegerOverflow=on  OutDataTypeStr=Inherit: Same as first input
  Switch15 : Switch  Threshold=1
  Switch16 : Switch  Threshold=Th
  Lvrt_time : Outport
  Lvrt : Outport  Port=2
  wires:
  Clock3/1 -> Sample and Hold3/1
  Sample and Hold3/1 -> Sum18/2
  Relay1/1 -> Lvrt/1, Scope/1, Divide2/2, Switch15/2, Sample and Hold3/Trigger
  Sum18/1 -> Switch15/1
  Switch16/1 -> Divide2/1
  " 3"/1 -> Switch16/3
  " 1"/1 -> Switch16/1
  Switch15/1 -> Switch16/2
  Clock6/1 -> Sum18/1
  " 1"/1 -> Switch15/3
  Divide2/1 -> Lvrt_time/1
  Ug/1 -> Relay1/1

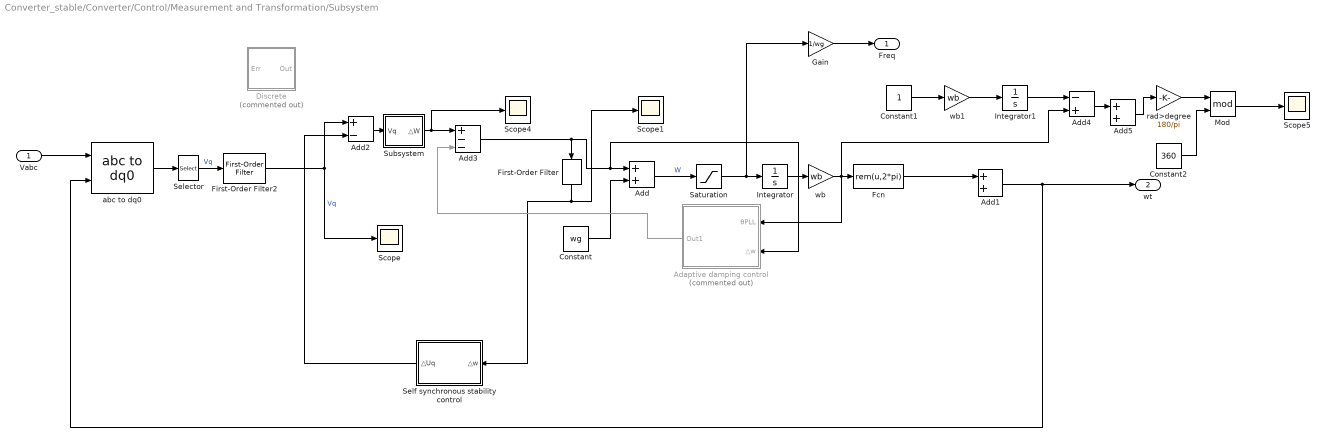
== system Converter_stable/Converter/Control/Measurement and Transformation/Subsystem ==
  Vabc : Inport  PortDimensions=3
  Adaptive damping control : Subsystem  Commented=on  mask{Vg=0.2, Lg=0.25, Id=0.8, thg=-90, znb=0.5}
      mask prompts: thg "θpcc"; znb "zu ni bi"
  Add : Sum
  Add1 : Sum
  Add2 : Sum  Inputs=+-
  Add3 : Sum  Inputs=+--
  Add4 : Sum  Inputs=-+
  Add5 : Sum
  Constant : Constant  Value=wg
  Constant1 : Constant
  Constant2 : Constant  Value=360
  Discrete : Subsystem  Commented=on  DialogController=POWERSYS.PowerSysDialog  VariantControl=PID_Discrete  mask(Discrete PID Controller){Kp=sps.Kp, Ki=sps.Ki, Kd=sps.Kd, TcD=sps.TcD, Par_Limits=[inf 0], Init=0, Ts=Ts}
      mask prompts: Kp "Proportional gain (Kp):"; Ki "Integral gain (Ki):"; Kd "Derivative gain (Kd):"; TcD "Time constant for derivative filter (s):"; Par_Limits "Output limits: [ Upper   Lower ]"; Init "Output initial value:"; Ts "Sample time:"
      mask help: This block implements a discrete PID controller.
      mask Display: disp('PID');
  Fcn : Fcn  Expr=rem(u,2*pi)
  First-Order Filter : spsFirstOrderFilterLib/First-Order Filter  FilterType=Lowpass  Tc=10e-3  Ts=Ts  Initialize=on  Vac_Init=[0, 0, 0]  Vdc_Init=0  PlotResponse=off  FreqRange="[0,  200,  1]"
  First-Order Filter2 : spsFirstOrderFilterLib/First-Order Filter  FilterType=Lowpass  Tc=10e-4  Ts=0  Initialize=on  Vac_Init=[0, 0, 50]  Vdc_Init=0  PlotResponse=off  FreqRange="[0,  200,  1]"
  Gain : Gain  Gain=1/wg
  Integrator : Integrator
  Integrator1 : Integrator
  Mod : Math  Operator=mod  SaturateOnIntegerOverflow=on
  Saturation : Saturate  UpperLimit=1.2*wg  LowerLimit=0.8*wg
  Scope{,1,4..5} (4 alike) : Scope
  Selector : Selector  InputPortWidth=3  IndexOptions=Index vector (dialog)  Indices=2  OutputSizes=1
  Self synchronous stability control : Subsystem  mask{kpr=1.2, kir=15, iq=0.75}
  Subsystem : Subsystem  mask(PI controller){}
      mask Display: disp('PI');
  abc to dq0 : spsabctodq0Lib/abc to dq0  Alignment=90 degrees behind phase A axis
  rad>degree : Gain  Gain=180/pi
  wb : Gain  Gain=wb
  wb1 : Gain  Gain=wb
  Freq : Outport  VectorParamsAs1DForOutWhenUnconnected=off
  wt : Outport  Port=2  VectorParamsAs1DForOutWhenUnconnected=off
  wires:
  abc to dq0/1 -> Selector/1
  Gain/1 -> Freq/1
  Vabc/1 -> abc to dq0/1
  Integrator/1 -> wb/1
  Add/1 -> Saturation/1  "W"
  wb/1 -> Adaptive damping control/1(θPLL), Fcn/1, Add4/2
  Constant/1 -> Add/2
  Saturation/1 -> Integrator/1, Gain/1
  Add3/1 -> Adaptive damping control/2(△w), Add/1, First-Order Filter/1
  Subsystem/1(△W) -> Scope4/1, Add3/1
  Fcn/1 -> Add1/1
  First-Order Filter2/1 -> Add2/1, Scope/1  "Vq"
  First-Order Filter/1 -> Scope1/1, Self synchronous stability control/1(△w)
  Add2/1 -> Subsystem/1(Vq)
  Self synchronous stability control/1(△Uq) -> Add2/2
  Selector/1 -> First-Order Filter2/1  "Vq"
  Add1/1 -> abc to dq0/2, wt/1
  Integrator1/1 -> Add4/1
  wb1/1 -> Integrator1/1
  Constant1/1 -> wb1/1
  Add5/1 -> rad>degree/1
  Mod/1 -> Scope5/1
  rad>degree/1 -> Mod/1
  Constant2/1 -> Mod/2
  Add4/1 -> Add5/1
  Adaptive damping control/1(Out1) -> Add3/3

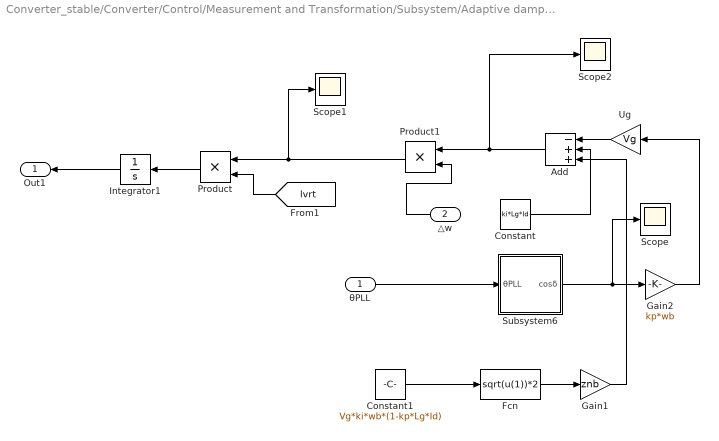
== system Converter_stable/Converter/Control/Measurement and Transformation/Subsystem/Adaptive damping control ==
  θPLL : Inport
  △w : Inport  Port=2
  Add : Sum  Inputs=-++
  Constant : Constant  Value=ki*Lg*Id
  Constant1 : Constant  Value=Vg*ki*wb*(1-kp*Lg*Id)
  Fcn : Fcn  Expr=sqrt(u(1))*2
  Gain1 : Gain  Gain=znb
  Gain2 : Gain  Gain=kp*wb
  Integrator1 : Integrator
  Product : Product
  Product1 : Product
  Scope : Scope
  Scope1 : Scope
  Scope2 : Scope
  Subsystem6 : Subsystem
  Ug : Gain  Gain=Vg
  Out1 : Outport
  wires:
  θPLL/1 -> Subsystem6/1(θPLL)
  Gain2/1 -> Ug/1
  Ug/1 -> Add/1
  Subsystem6/1(cosδ) -> Scope/1, Gain2/1
  Product1/1 -> Scope1/1, Product/1
  Add/1 -> Scope2/1, Product1/1
  Constant/1 -> Add/2
  Integrator1/1 -> Out1/1
  [lvrt] -> Product/2
  △w/1 -> Product1/2
  Product/1 -> Integrator1/1
  Constant1/1 -> Fcn/1
  Fcn/1 -> Gain1/1
  Gain1/1 -> Add/3

== system Converter_stable/Converter/Control/Measurement and Transformation/Subsystem/Discrete ==
  Err : Inport  SampleTime=Ts
  "Discrete Derivative " : DiscreteTransferFcn  Numerator="[ 1  -1 ]*Kd"  Denominator="[ TcD  Ts-TcD ]"  SampleTime=Ts
  Discrete-Time Integrator : DiscreteIntegrator  gainval=Ki  InitialCondition=Init  SampleTime=Ts  LimitOutput=on  UpperSaturationLimit=Par_Limits(1)  LowerSaturationLimit=Par_Limits(2)  ICPrevOutput=DiscIntNeverNeededParam  ICPrevScaledInput=DiscIntNeverNeededParam
  Kp4 : Gain  Gain=Kp  SaturateOnIntegerOverflow=on  SampleTime=Ts  OutDataTypeStr=Inherit: Same as input  ParamDataTypeStr=Inherit: Same as input
  Saturation1 : Saturate  UpperLimit=Par_Limits(1)  LowerLimit=Par_Limits(2)  SampleTime=Ts
  Sum6 : Sum  Inputs=+++  InputSameDT=on  SaturateOnIntegerOverflow=on  SampleTime=Ts  OutDataTypeStr=Inherit: Same as first input
  Out : Outport  SampleTime=Ts  InitialOutput=0  VectorParamsAs1DForOutWhenUnconnected=off
  wires:
  Saturation1/1 -> Out/1
  Err/1 -> "Discrete Derivative "/1, Discrete-Time Integrator/1, Kp4/1
  Sum6/1 -> Saturation1/1
  Kp4/1 -> Sum6/1
  Discrete-Time Integrator/1 -> Sum6/2
  "Discrete Derivative "/1 -> Sum6/3

== system Converter_stable/Converter/Control/Measurement and Transformation/Subsystem/Self synchronous stability control ==
  △w : Inport
  Product : Product
  Product1 : Product
  Subsystem4 : Subsystem  mask(PI controller){}
      mask Display: disp('PI');
  wb3 : Gain  Gain=iq
  △Uq : Outport
  wires:
  Product1/1 -> △Uq/1
  [lvrt] -> Product1/1
  [lvrt] -> Product/2
  Product/1 -> Subsystem4/1(Vq)
  wb3/1 -> Product1/2
  Subsystem4/1(△W) -> wb3/1
  △w/1 -> Product/1

== system Converter_stable/Converter/Control/Measurement and Transformation/Subsystem/Subsystem ==
  Vq : Inport
  Add3 : Sum
  Gain2 : Gain  Gain=ki
  Gain3 : Gain  Gain=kp
  Integrator1 : Integrator
  Saturation : Saturate  Commented=on  UpperLimit=0.2*wg  LowerLimit=-0.2*wg
  △W : Outport
  wires:
  Vq/1 -> Gain3/1, Gain2/1
  Gain2/1 -> Integrator1/1
  Integrator1/1 -> Add3/2
  Add3/1 -> △W/1  "△W"
  Gain3/1 -> Add3/1

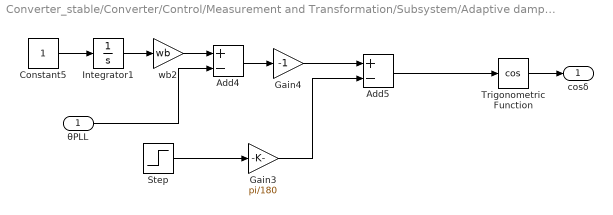
== system Converter_stable/Converter/Control/Measurement and Transformation/Subsystem/Adaptive damping control/Subsystem6 ==
  θPLL : Inport
  Add4 : Sum  Inputs=+-
  Add5 : Sum  Inputs=+-
  Constant5 : Constant
  Gain3 : Gain  Gain=pi/180
  Gain4 : Gain  Gain=-1
  Integrator1 : Integrator
  Step : Step  Time=0.6  After=thg  SampleTime=0
  Trigonometric Function : Trigonometry  Operator=cos
  wb2 : Gain  Gain=wb
  cosδ : Outport
  wires:
  θPLL/1 -> Add4/2
  wb2/1 -> Add4/1
  Gain3/1 -> Add5/2
  Integrator1/1 -> wb2/1
  Add4/1 -> Gain4/1
  Constant5/1 -> Integrator1/1
  Add5/1 -> Trigonometric Function/1
  Step/1 -> Gain3/1
  Gain4/1 -> Add5/1
  Trigonometric Function/1 -> cosδ/1

== system Converter_stable/Converter/Control/Measurement and Transformation/Subsystem/Self synchronous stability control/Subsystem4 ==
  Vq : Inport
  Add3 : Sum
  Gain2 : Gain  Gain=kir
  Gain3 : Gain  Gain=kpr
  Integrator1 : Integrator
  Saturation : Saturate  Commented=on  UpperLimit=0.2*wg  LowerLimit=-0.2*wg
  △W : Outport
  wires:
  Vq/1 -> Gain3/1, Gain2/1
  Gain2/1 -> Integrator1/1
  Integrator1/1 -> Add3/2
  Add3/1 -> △W/1  "△W"
  Gain3/1 -> Add3/1
